simulink model "unit_and_array_doubleRx"  (R2019b)
settings: Solver=VariableStepAuto  StartTime=0.0  StopTime=0.0005  RelTol=1e-3
libraries: fl_lib x24, nesl_utility x12, ee_lib x6, powerlib_meascontrol x2
settings Model: Creator=LRF  LastModifiedBy=LRF

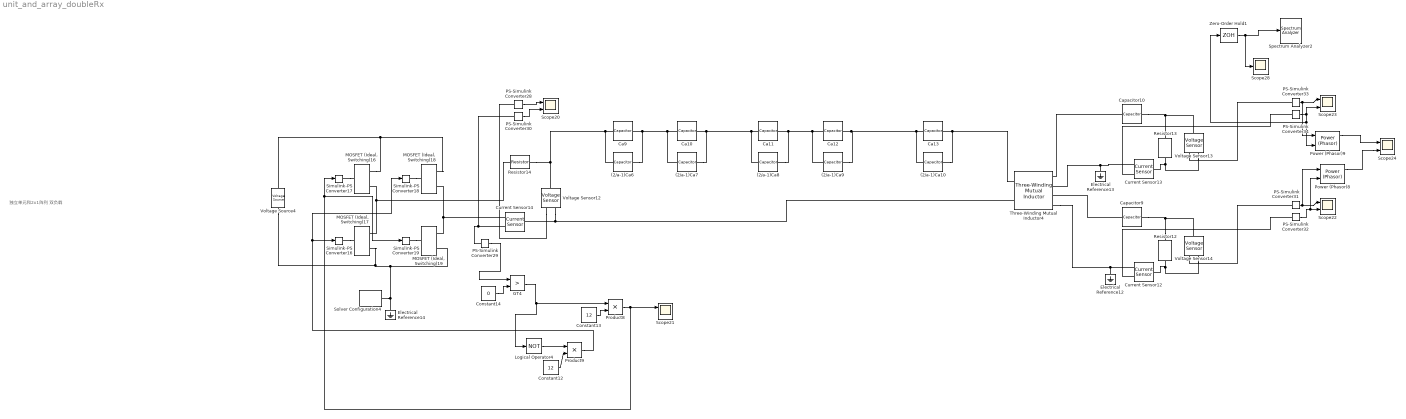
== system unit_and_array_doubleRx ==
  note: 独立单元和2x1阵列 双负载
  (2/a-1)Ca{6..10} (5 alike) : fl_lib/Electrical/Electrical Elements/Capacitor  c=379 pF  r=1e-6 Ohm  g=0 1/Ohm  i_specify=off  i_priority=None  i=0 A  i_nominal_specify=off  i_nominal_unit=A  i_nominal_value=1  v_specify=off  v_priority=None  v=0 V  v_nominal_specify=off  v_nominal_unit=V  v_nominal_value=1  vc_specify=off  vc_priority=High  vc=0 V  vc_nominal_specify=off  vc_nominal_unit=V  vc_nominal_value=1
  Ca{9..13} (5 alike) : fl_lib/Electrical/Electrical Elements/Capacitor  c=1517 pF  r=1e-6 Ohm  g=0 1/Ohm  i_specify=off  i_priority=None  i=0 A  i_nominal_specify=off  i_nominal_unit=A  i_nominal_value=1  v_specify=off  v_priority=None  v=0 V  v_nominal_specify=off  v_nominal_unit=V  v_nominal_value=1  vc_specify=off  vc_priority=High  vc=0 V  vc_nominal_specify=off  vc_nominal_unit=V  vc_nominal_value=1
  Capacitor10 : fl_lib/Electrical/Electrical Elements/Capacitor  c=1013 pF  r=1e-6 Ohm  g=0 1/Ohm  i_specify=off  i_priority=None  i=0 A  i_nominal_specify=off  i_nominal_unit=A  i_nominal_value=1  v_specify=off  v_priority=None  v=0 V  v_nominal_specify=off  v_nominal_unit=V  v_nominal_value=1  vc_specify=off  vc_priority=High  vc=0 V  vc_nominal_specify=off  vc_nominal_unit=V  vc_nominal_value=1
  Capacitor9 : fl_lib/Electrical/Electrical Elements/Capacitor  c=1013 pF  r=1e-6 Ohm  g=0 1/Ohm  i_specify=off  i_priority=None  i=0 A  i_nominal_specify=off  i_nominal_unit=A  i_nominal_value=1  v_specify=off  v_priority=None  v=0 V  v_nominal_specify=off  v_nominal_unit=V  v_nominal_value=1  vc_specify=off  vc_priority=High  vc=0 V  vc_nominal_specify=off  vc_nominal_unit=V  vc_nominal_value=1
  Constant12 : Constant  Value=12
  Constant13 : Constant  Value=12
  Constant14 : Constant  Value=0
  Current Sensor12 : fl_lib/Electrical/Electrical Sensors/Current Sensor
  Current Sensor13 : fl_lib/Electrical/Electrical Sensors/Current Sensor
  Current Sensor14 : fl_lib/Electrical/Electrical Sensors/Current Sensor
  Electrical Reference12 : fl_lib/Electrical/Electrical Elements/Electrical Reference
  Electrical Reference13 : fl_lib/Electrical/Electrical Elements/Electrical Reference
  Electrical Reference14 : fl_lib/Electrical/Electrical Elements/Electrical Reference
  GT4 : RelationalOperator  Operator=>  OutDataTypeStr=boolean  RndMeth=Simplest
  Logical Operator4 : Logic  Operator=NOT  AllPortsSameDT=off  OutDataTypeStr=boolean
  MOSFET (Ideal, Switching){16..19} (4 alike) : ee_lib/Semiconductors & Converters/MOSFET (Ideal, Switching)  Rds=0.01 Ohm  Goff=1e-6 1/Ohm  Vth=2 V  diode_param=1  diode_Vf=0.8 V  diode_Ron=0.001 Ohm  diode_Goff=1e-5 1/Ohm  diode_C=50e-9 F  diode_iRM=-235 A  diode_iF=300 A  diode_idot=-50 A/us  diode_trr_param=1  diode_trr_factor=3  diode_trr=15 us  diode_Qrr=1500 s*uA  thermal_loss_option=2  Voff=300 V  Tau=1e-4 s  Tj=[298.15, 398.15] K  Iout_scalar=600 A  Eon_scalar=22.86e-3 J  Eoff_scalar=17.14e-3 J  Von_scalar=2.7 V  Iout_data=[0, 10, 50, 100, 200, 400, 600] A  Eon_data=[0, .29, 1.43, 2.86, 5.71, 13.14, 22.86; 0, .57, 2.63, 5.14, 10.29, 20.57, 30.29] * 1e-3 J  Eoff_data=[0, .21, 1.07, 2.14, 4.29, 9.86, 17.14; 0, .43, 1.97, 3.86, 7.71, 15.43, 22.71] * 1e-3 J  Von_data=[0, 1.1, 1.3, 1.45, 1.75, 2.25, 2.7; 0, 1, 1.15, 1.35, 1.7, 2.35, 3] V
      settings: SourceProductName=Simscape Electrical
  PS-Simulink Converter{28..34} (7 alike) : nesl_utility/PS-Simulink Converter  PhysicalDomain=network_engine_domain  SubClassName=ps_output  LeftPortType=input  RightPortType=output  PseudoPeriodic=off  Frequencies=[]  Unit=inherit  AffineConversion=off
  Power (Phasor)8 : powerlib_meascontrol/Measurements/Power (Phasor)
      settings: SourceProductName=Simscape Electrical  SourceProductBaseCode=PS
  Power (Phasor)9 : powerlib_meascontrol/Measurements/Power (Phasor)
      settings: SourceProductName=Simscape Electrical  SourceProductBaseCode=PS
  Product8 : Product
  Product9 : Product
  Resistor12 : fl_lib/Electrical/Electrical Elements/Resistor  R=15 Ohm  i_specify=off  i_priority=None  i=0 A  i_nominal_specify=off  i_nominal_unit=A  i_nominal_value=1  v_specify=off  v_priority=None  v=0 V  v_nominal_specify=off  v_nominal_unit=V  v_nominal_value=1
  Resistor13 : fl_lib/Electrical/Electrical Elements/Resistor  R=15 Ohm  i_specify=off  i_priority=None  i=0 A  i_nominal_specify=off  i_nominal_unit=A  i_nominal_value=1  v_specify=off  v_priority=None  v=0 V  v_nominal_specify=off  v_nominal_unit=V  v_nominal_value=1
  Resistor14 : fl_lib/Electrical/Electrical Elements/Resistor  R=0 Ohm  i_specify=off  i_priority=None  i=0 A  i_nominal_specify=off  i_nominal_unit=A  i_nominal_value=1  v_specify=off  v_priority=None  v=0 V  v_nominal_specify=off  v_nominal_unit=V  v_nominal_value=1
  Scope{20..24} (5 alike) : Scope  NumInputPorts=2
  Scope28 : Scope
  Simulink-PS Converter{16..19} (4 alike) : nesl_utility/Simulink-PS Converter  PhysicalDomain=network_engine_domain  SubClassName=ps_input  LeftPortType=input  RightPortType=output  PseudoPeriodic=off  Frequencies=[]  NoiseDistribution=none  NoiseParameters=[]  Unit=1  AffineConversion=off  FilteringAndDerivatives=provide  SimscapeFilterOrder=1  InputFilterTimeConstant=0.001  UdotUserProvided=0
  Solver Configuration4 : nesl_utility/Solver Configuration  PhysicalDomain=network_engine_domain  SubClassName=solver  LeftPortType=input  RightPortType=generic  Tones=[]  Harmonics=[]  SimulateNoise=off  Profile=off  UseLocalSampling=off  EnableSwitchedLinearOptims=on  FrequencyDomain=off  UseCCode=off  RelTol=0.001  AbsTol=1e-06  MinStep=1e-09  ToWorkspace=off  RevertToSquareIcSolve=off  NumHomotopyIterations=100  PhasorMode=off  PhasorModeNumHarmonics=1  DoDC=off  ResidualTolerance=1e-09  UseLocalSolver=off  LocalSolverChoice=NE_BACKWARD_EULER_ADVANCER  LocalSolverSampleTime=0.001  DoFixedCost=off  MaxNonlinIter=3  MaxModeIter=2  LinearAlgebra=auto  EquationFormulation=NE_TIME_EF  DelaysMemoryBudget=1024  AutomaticFiltering=on  FilteringTimeConstant=0.001  PartitionStorageMethod=AS_NEEDED  PartitionMemoryBudget=1024  PartitionMethod=ROBUST
  Spectrum Analyzer2 : SpectrumAnalyzer
  Three-Winding Mutual Inductor4 : ee_lib/Passive/Transformers/Three-Winding Mutual Inductor  L1=280.67 uH  L2=100 uH  L3=100 uH  K12=0.1  K13=0.1  K23=0  IC_given=1  IC1=0 A  IC2=0 A  IC3=0 A
      settings: SourceProductName=Simscape Electrical  SourceProductBaseCode=PS  InternalSimscapePortConfiguration="{\"Bottom\":[],\"Left\":[{\"id\":\"p1\",\"label\":\"1+\",\"type\":\"foundation.electrical.electrical\"},{\"id\":\"n1\",\"label\":\"1-\",\"type\":\"foundation.electrical.electrical\"}],\"Right\":[{\"id\":\"p2\",\"label\":\"2+\",\"type\":\"foundation.electrical.electrical\"},{\"id\":\"n2\",\"label\":\"2-\",\"type\":\"foundation.electrical.electrical\"},{\"id\":\"p3\",\"label\":\"3+\",\"type\":\"foundation.electrical.electrical\"},{\"id\":\"n3\",\"label\":\"3-\",\"type\":\"foundation.electrical.electrical\"}],\"Top\":[]}"
  Voltage Sensor12 : fl_lib/Electrical/Electrical Sensors/Voltage Sensor
  Voltage Sensor13 : fl_lib/Electrical/Electrical Sensors/Voltage Sensor
  Voltage Sensor14 : fl_lib/Electrical/Electrical Sensors/Voltage Sensor
  Voltage Source4 : ee_lib/Sources/Voltage Source  dc_voltage=15 V  ac_voltage=0 V  ac_shift=0 rad  ac_frequency=60 Hz  noise_mode=0  PSD=0 V^2/Hz  repeatability=1  auto_seed=170723637  user_seed=0  sample_time=1e-3 s  i_specify=off  i_priority=None  i=0 A  i_nominal_specify=off  i_nominal_unit=A  i_nominal_value=1  v_specify=off  v_priority=None  v=0 V  v_nominal_specify=off  v_nominal_unit=V  v_nominal_value=1
      settings: SourceProductName=Simscape Electrical
  Zero-Order Hold1 : ZeroOrderHold  SampleTime=1e-7
  wires:
  PS-Simulink Converter33/1 -> Power (Phasor)9/1, Scope23/1
  PS-Simulink Converter32/1 -> Power (Phasor)8/2, Scope22/2
  Logical Operator4/1 -> Product9/1
  Constant13/1 -> Product8/2
  Product8/1 -> Simulink-PS Converter19/1, Simulink-PS Converter17/1, Scope21/1
  Product9/1 -> Simulink-PS Converter18/1, Simulink-PS Converter16/1
  Power (Phasor)9/1 -> Scope24/1
  PS-Simulink Converter31/1 -> Power (Phasor)8/1, Scope22/1
  Constant12/1 -> Product9/2
  Power (Phasor)8/1 -> Scope24/2
  GT4/1 -> Logical Operator4/1, Product8/1
  Constant14/1 -> GT4/2
  PS-Simulink Converter28/1 -> Scope20/1
  PS-Simulink Converter30/1 -> Scope20/2
  PS-Simulink Converter29/1 -> GT4/1
  Zero-Order Hold1/1 -> Scope28/1, Spectrum Analyzer2/1
  PS-Simulink Converter34/1 -> Power (Phasor)9/2, Zero-Order Hold1/1, Scope23/2
  connections:
  Voltage Sensor12/LConn1 -- Resistor14/RConn1 -- (2/a-1)Ca6/LConn1 -- Ca9/LConn1
  Resistor12/RConn1 -- Voltage Sensor14/RConn2 -- Current Sensor12/LConn1
  "MOSFET (Ideal, Switching)19"/RConn2 -- Solver Configuration4/RConn1 -- Electrical Reference14/LConn1 -- "MOSFET (Ideal, Switching)17"/RConn2 -- Voltage Source4/RConn1
  Current Sensor14/LConn1 -- Voltage Sensor12/RConn2 -- Three-Winding Mutual Inductor4/LConn2
  Resistor12/LConn1 -- Capacitor9/RConn1 -- Voltage Sensor14/LConn1
  Voltage Sensor13/LConn1 -- Resistor13/LConn1 -- Capacitor10/RConn1
  "MOSFET (Ideal, Switching)18"/RConn1 -- "MOSFET (Ideal, Switching)16"/RConn1 -- Voltage Source4/LConn1
  Ca10/LConn1 -- (2/a-1)Ca7/LConn1 -- (2/a-1)Ca6/RConn1 -- Ca9/RConn1
  Three-Winding Mutual Inductor4/RConn2 -- Current Sensor13/RConn2 -- Electrical Reference13/LConn1
  Resistor14/LConn1 -- "MOSFET (Ideal, Switching)17"/RConn1 -- "MOSFET (Ideal, Switching)16"/RConn2
  Ca12/LConn1 -- (2/a-1)Ca9/LConn1 -- (2/a-1)Ca8/RConn1 -- Ca11/RConn1
  Current Sensor12/RConn2 -- Electrical Reference12/LConn1 -- Three-Winding Mutual Inductor4/RConn4
  Current Sensor13/LConn1 -- Resistor13/RConn1 -- Voltage Sensor13/RConn2
  PS-Simulink Converter29/LConn1 -- Current Sensor14/RConn1 -- PS-Simulink Converter30/LConn1
  (2/a-1)Ca10/LConn1 -- Ca12/RConn1 -- (2/a-1)Ca9/RConn1 -- Ca13/LConn1
  (2/a-1)Ca7/RConn1 -- Ca11/LConn1 -- (2/a-1)Ca8/LConn1 -- Ca10/RConn1
  "MOSFET (Ideal, Switching)18"/RConn2 -- "MOSFET (Ideal, Switching)19"/RConn1 -- Current Sensor14/RConn2
  PS-Simulink Converter33/LConn1 -- Voltage Sensor13/RConn1
  Voltage Sensor12/RConn1 -- PS-Simulink Converter28/LConn1
  Capacitor9/LConn1 -- Three-Winding Mutual Inductor4/RConn3
  Current Sensor12/RConn1 -- PS-Simulink Converter32/LConn1
  Capacitor10/LConn1 -- Three-Winding Mutual Inductor4/RConn1
  Current Sensor13/RConn1 -- PS-Simulink Converter34/LConn1
  Simulink-PS Converter18/RConn1 -- "MOSFET (Ideal, Switching)18"/LConn1
  Simulink-PS Converter16/RConn1 -- "MOSFET (Ideal, Switching)17"/LConn1
  PS-Simulink Converter31/LConn1 -- Voltage Sensor14/RConn1
  Simulink-PS Converter19/RConn1 -- "MOSFET (Ideal, Switching)19"/LConn1
  Simulink-PS Converter17/RConn1 -- "MOSFET (Ideal, Switching)16"/LConn1
  (2/a-1)Ca10/RConn1 -- Ca13/RConn1 -- Three-Winding Mutual Inductor4/LConn1
